simulink model "platoon_project"  (Simulink 8.9)
settings: Solver=FixedStepAuto  StartTime=0.0  StopTime=5  FixedStep=0.1  RelTol=1e-3  EnableMultiTasking=on
model workspace (MAT data in the model file):
  Kd_brake = 0
  Kd_throttle = 0
  Ki_brake = 1
  Ki_throttle = 1
  Kp_brake = 5000
  Kp_throttle = 15
  L : num (value not decoded)
values from neighbouring files (symbols this model uses):
  tnet_table = [57.5127074443 119.897368421 182.282029398 223.675296349 261.549751738 274.206057597 279.305263158 283.689473684 288.073684211 292.467532318 296.875779086 301.284025854 ... (400 elements, 20x20)]    [enginemap.mat]    (also in genmap.m = griddata(map_ford(:,1), map_ford(:,4), map_ford(:,2), we_tab)
  we_max = 471.2    [enginemap.mat]    (also in genmap.m = max(map_ford(:,1)))
  we_min = 57.6    [enginemap.mat]    (also in genmap.m = min(map_ford(:,1)))
undefined symbols (not defined in the file or in its folder): c_aero, delay_brake, F_roll, h, I_e, I_wheel, KB, mass, max_throttle, max_throttle_rate, min_throttle, mu_B, mu_C, mu_D, mu_E, P_po, Rdrive, tau_brake, tau_throttle, throttle_o, w_wheel_o, we_o, x_dot_o
libraries: simulink x10
(part 1 of 3)
settings Model: Creator=user  LastModifiedBy=edward
settings OptimizationCC: ExpressionDepthLimit=2147483647  InitFltsAndDblsToZero=on
settings DebuggingCC: SolverPrmCheckMsg=warning  FcnCallInpInsideContextMsg=error
settings GRTTargetCC: GeneratePreprocessorConditionals=Use local settings

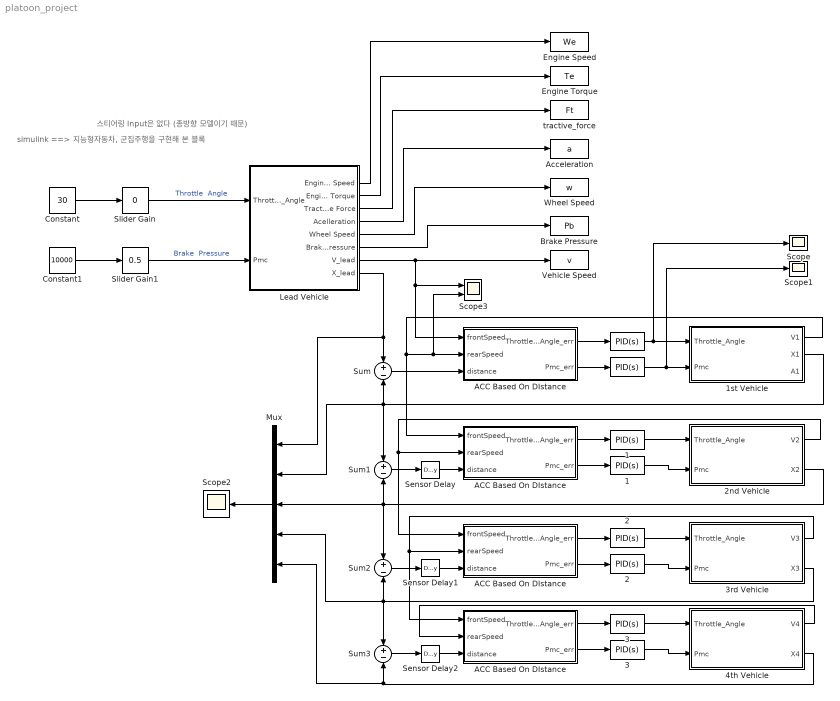
== system platoon_project ==
  note: simulink ==> 지능형자동차, 군집주행을 구현해 본 블록
  note: 스티어링 Input은 없다 (종방향 모델이기 때문)
   {,1..3} (4 alike) : simulink/Continuous/PID Controller  Controller=PID  TimeDomain=Continuous-time  SampleTime=-1  IntegratorMethod=Forward Euler  FilterMethod=Forward Euler  Form=Parallel  UseFilter=on  ControllerParametersSource=internal  P=Kp_throttle  I=Ki_throttle  D=Kd_throttle  N=100  InitialConditionSource=internal  InitialConditionForIntegrator=0  InitialConditionForFilter=0  ExternalReset=none  LimitOutput=off  UpperSaturationLimit=inf  LowerSaturationLimit=-inf  LinearizeAsGain=on  AntiWindupMode=none  Kb=1  TrackingMode=off  Kt=1  PParamMin=[]  PParamMax=[]  IParamMin=[]  IParamMax=[]  DParamMin=[]  DParamMax=[]  NParamMin=[]  NParamMax=[]  KbParamMin=[]  KbParamMax=[]  KtParamMin=[]  KtParamMax=[]  POutMin=[]  POutMax=[]  IOutMin=[]  IOutMax=[]  DOutMin=[]  DOutMax=[]  NOutMin=[]  NOutMax=[]  KbOutMin=[]  KbOutMax=[]  KtOutMin=[]  KtOutMax=[]  IntegratorOutMin=[]  IntegratorOutMax=[]  FilterOutMin=[]  FilterOutMax=[]  SumOutMin=[]  SumOutMax=[]  SumI1OutMin=[]  SumI1OutMax=[]  SumI2OutMin=[]  SumI2OutMax=[]  SumI3OutMin=[]  SumI3OutMax=[]  SumDOutMin=[]  SumDOutMax=[]  SaturationOutMin=[]  SaturationOutMax=[]  IntegratorContinuousStateAttributes=''  IntegratorStateMustResolveToSignalObject=off  IntegratorRTWStateStorageClass=Auto  FilterContinuousStateAttributes=''  FilterStateMustResolveToSignalObject=off  FilterRTWStateStorageClass=Auto  DifferentiatorICPrevScaledInput=0  DifferentiatorOutMin=[]  DifferentiatorOutMax=[]  InitialConditionSetting=State (most efficient)
    {,1..3} (4 alike) : simulink/Continuous/PID Controller  Controller=PID  TimeDomain=Continuous-time  SampleTime=-1  IntegratorMethod=Forward Euler  FilterMethod=Forward Euler  Form=Parallel  UseFilter=on  ControllerParametersSource=internal  P=Kp_brake  I=Ki_brake  D=Kd_brake  N=100  InitialConditionSource=internal  InitialConditionForIntegrator=0  InitialConditionForFilter=0  ExternalReset=none  LimitOutput=off  UpperSaturationLimit=inf  LowerSaturationLimit=-inf  LinearizeAsGain=on  AntiWindupMode=none  Kb=1  TrackingMode=off  Kt=1  PParamMin=[]  PParamMax=[]  IParamMin=[]  IParamMax=[]  DParamMin=[]  DParamMax=[]  NParamMin=[]  NParamMax=[]  KbParamMin=[]  KbParamMax=[]  KtParamMin=[]  KtParamMax=[]  POutMin=[]  POutMax=[]  IOutMin=[]  IOutMax=[]  DOutMin=[]  DOutMax=[]  NOutMin=[]  NOutMax=[]  KbOutMin=[]  KbOutMax=[]  KtOutMin=[]  KtOutMax=[]  IntegratorOutMin=[]  IntegratorOutMax=[]  FilterOutMin=[]  FilterOutMax=[]  SumOutMin=[]  SumOutMax=[]  SumI1OutMin=[]  SumI1OutMax=[]  SumI2OutMin=[]  SumI2OutMax=[]  SumI3OutMin=[]  SumI3OutMax=[]  SumDOutMin=[]  SumDOutMax=[]  SaturationOutMin=[]  SaturationOutMax=[]  IntegratorContinuousStateAttributes=''  IntegratorStateMustResolveToSignalObject=off  IntegratorRTWStateStorageClass=Auto  FilterContinuousStateAttributes=''  FilterStateMustResolveToSignalObject=off  FilterRTWStateStorageClass=Auto  DifferentiatorICPrevScaledInput=0  DifferentiatorOutMin=[]  DifferentiatorOutMax=[]  InitialConditionSetting=State (most efficient)
  "                ACC Based On DIstance           " : MATLAB Function  TreatAsAtomicUnit=on
  "               ACC Based On DIstance           " : MATLAB Function  TreatAsAtomicUnit=on
  "               ACC Based On DIstance            " : MATLAB Function  TreatAsAtomicUnit=on
  "               ACC Based On DIstance             " : MATLAB Function  TreatAsAtomicUnit=on
  1st Vehicle : Subsystem
  2nd Vehicle : Subsystem
  3rd Vehicle : Subsystem
  4th Vehicle : Subsystem
  Acceleration : ToWorkspace  VariableName=a  SampleTime=-1
  Brake Pressure : ToWorkspace  VariableName=Pb  SampleTime=-1
  Constant : Constant  Value=30
  Constant1 : Constant  Value=10000
  Engine Speed : ToWorkspace  VariableName=We  SampleTime=-1
  Engine Torque : ToWorkspace  VariableName=Te  SampleTime=-1
  Lead Vehicle : Subsystem
  Mux : Mux  Inputs=5
  Scope : Scope
  Scope1 : Scope
  Scope2 : Scope
  Scope3 : Scope  NumInputPorts=2
  Sensor Delay : TransportDelay  DelayTime=0.1
  Sensor Delay1 : TransportDelay  DelayTime=0.2
  Sensor Delay2 : TransportDelay  DelayTime=0.3
  Slider Gain : simulink/Math Operations/Slider Gain  gain=0  low=0  high=1
  Slider Gain1 : simulink/Math Operations/Slider Gain  gain=0.5  low=0  high=1
  Sum{,1..3} (4 alike) : Sum  Inputs=+|-
  Vehicle Speed : ToWorkspace  VariableName=v  SampleTime=-1
  Wheel Speed : ToWorkspace  VariableName=w  SampleTime=-1
  tractive_force : ToWorkspace  VariableName=Ft  SampleTime=-1
  wires:
  Constant/1 -> Slider Gain/1
  Slider Gain/1 -> Lead Vehicle/1(Throttle_Angle)  "Throttle  Angle"
  Constant1/1 -> Slider Gain1/1
  Slider Gain1/1 -> Lead Vehicle/2(Pmc)  "Brake  Pressure"
  Lead Vehicle/1(Engine Speed) -> Engine Speed/1
  Lead Vehicle/3(Tractive Force) -> tractive_force/1
  Lead Vehicle/4(Acelleration) -> Acceleration/1
  Lead Vehicle/5(Wheel Speed) -> Wheel Speed/1
  Lead Vehicle/6(Brake Pressure) -> Brake Pressure/1
  Lead Vehicle/2(Engine Torque) -> Engine Torque/1
  Lead Vehicle/8(X_lead) -> Mux/1, Sum/1
  1st Vehicle/2(X1) -> Mux/2, Sum1/1, Sum/2
  Sum/1 -> "               ACC Based On DIstance           "/3(distance)
  Lead Vehicle/7("V_lead ") -> "               ACC Based On DIstance           "/1(frontSpeed), Scope3/1, Vehicle Speed/1
  1st Vehicle/1(V1) -> "               ACC Based On DIstance            "/1(frontSpeed), Scope3/2, "               ACC Based On DIstance           "/2(rearSpeed)
  2nd Vehicle/2(X2) -> Mux/3, Sum2/1, Sum1/2
  2nd Vehicle/1(V2) -> "                ACC Based On DIstance           "/1(frontSpeed), "               ACC Based On DIstance            "/2(rearSpeed)
  Sum1/1 -> Sensor Delay/1
  "               ACC Based On DIstance           "/1(Throttle_Angle_err) -> " "/1
  "               ACC Based On DIstance           "/2(Pmc_err) -> "  "/1
  " "/1 -> Scope/1, 1st Vehicle/1(Throttle_Angle)
  " 1"/1 -> 2nd Vehicle/1(Throttle_Angle)
  "               ACC Based On DIstance            "/2(Pmc_err) -> "  1"/1
  "               ACC Based On DIstance            "/1(Throttle_Angle_err) -> " 1"/1
  "  1"/1 -> 2nd Vehicle/2(Pmc)
  "  2"/1 -> 3rd Vehicle/2(Pmc)
  " 2"/1 -> 3rd Vehicle/1(Throttle_Angle)
  "                ACC Based On DIstance           "/1(Throttle_Angle_err) -> " 2"/1
  "                ACC Based On DIstance           "/2(Pmc_err) -> "  2"/1
  " 3"/1 -> 4th Vehicle/1(Throttle_Angle)
  "  3"/1 -> 4th Vehicle/2(Pmc)
  "               ACC Based On DIstance             "/1(Throttle_Angle_err) -> " 3"/1
  "               ACC Based On DIstance             "/2(Pmc_err) -> "  3"/1
  3rd Vehicle/2(X3) -> Mux/4, Sum3/1, Sum2/2
  Sum2/1 -> Sensor Delay1/1
  3rd Vehicle/1(V3) -> "               ACC Based On DIstance             "/1(frontSpeed), "                ACC Based On DIstance           "/2(rearSpeed)
  4th Vehicle/2(X4) -> Mux/5, Sum3/2
  Sum3/1 -> Sensor Delay2/1
  4th Vehicle/1(V4) -> "               ACC Based On DIstance             "/2(rearSpeed)
  Sensor Delay/1 -> "               ACC Based On DIstance            "/3(distance)
  Sensor Delay1/1 -> "                ACC Based On DIstance           "/3(distance)
  Sensor Delay2/1 -> "               ACC Based On DIstance             "/3(distance)
  "  "/1 -> Scope1/1, 1st Vehicle/2(Pmc)
  Mux/1 -> Scope2/1

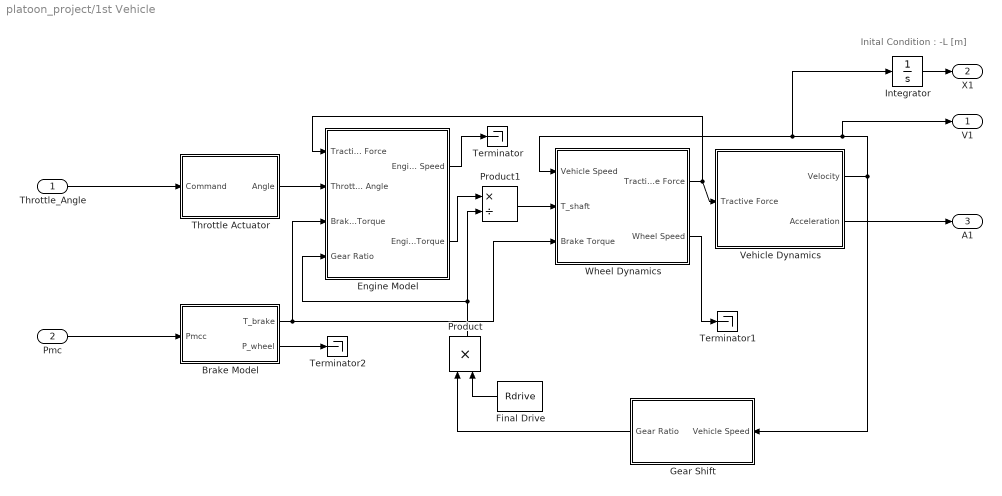
== system platoon_project/1st Vehicle ==
  note: Inital Condition : -L [m]
  Throttle_Angle : Inport
  Pmc : Inport  Port=2
  Brake Model : Subsystem
  Engine Model : Subsystem
  Final Drive : Constant  Value=Rdrive
  Gear Shift : Subsystem
  Integrator : Integrator  InitialCondition=-L
  Product : Product  Inputs=**  SaturateOnIntegerOverflow=on  RndMeth=Zero  InputSameDT=on  OutDataTypeStr=Inherit: Same as first input
  Product1 : Product  Inputs=*/  SaturateOnIntegerOverflow=on  RndMeth=Zero  InputSameDT=on  OutDataTypeStr=Inherit: Same as first input
  Terminator : Terminator
  Terminator1 : Terminator
  Terminator2 : Terminator
  Throttle Actuator : Subsystem
  Vehicle Dynamics : Subsystem
  Wheel Dynamics : Subsystem
  V1 : Outport
  X1 : Outport  Port=2
  A1 : Outport  Port=3
  wires:
  Vehicle Dynamics/1(Velocity) -> Gear Shift/1(Vehicle Speed), V1/1, Integrator/1, Wheel Dynamics/1(Vehicle Speed)
  Pmc/1 -> Brake Model/1(Pmcc)
  Throttle_Angle/1 -> Throttle Actuator/1(Command)
  Throttle Actuator/1(Angle) -> Engine Model/2(Throttle Angle)
  Wheel Dynamics/1(Tractive Force) -> Engine Model/1(Tractive Force), Vehicle Dynamics/1(Tractive Force)
  Gear Shift/1(Gear Ratio) -> Product/1
  Final Drive/1 -> Product/2
  Product/1 -> Engine Model/4(Gear Ratio), Product1/2
  Brake Model/1(T_brake) -> Wheel Dynamics/3(Brake Torque), Engine Model/3(Brake Torque)
  Engine Model/2(Engine Torque) -> Product1/1
  Product1/1 -> Wheel Dynamics/2(T_shaft)
  Engine Model/1(Engine Speed) -> Terminator/1
  Wheel Dynamics/2(Wheel Speed) -> Terminator1/1
  Brake Model/2(P_wheel) -> Terminator2/1
  Vehicle Dynamics/2(Acceleration) -> A1/1
  Integrator/1 -> X1/1

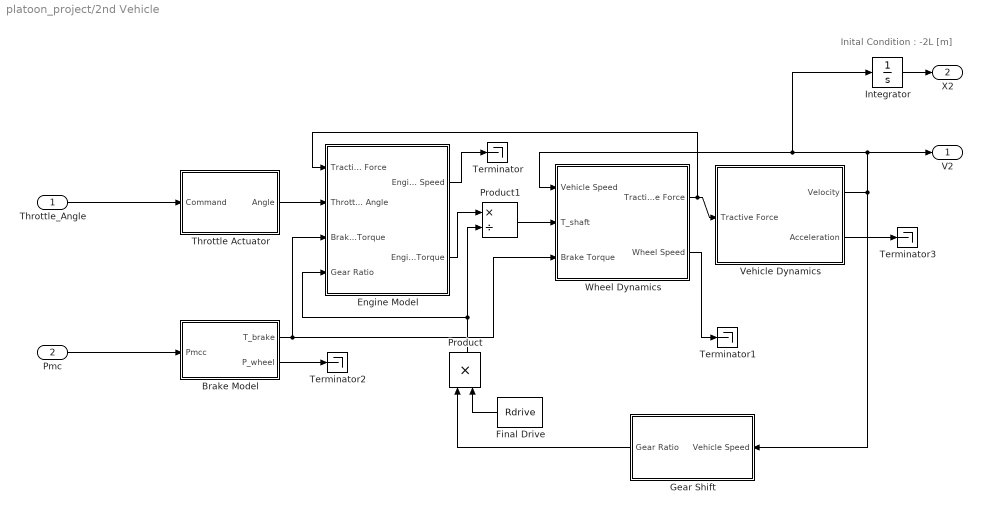
== system platoon_project/2nd Vehicle ==
  note: Inital Condition : -2L [m]
  Throttle_Angle : Inport
  Pmc : Inport  Port=2
  Brake Model : Subsystem
  Engine Model : Subsystem
  Final Drive : Constant  Value=Rdrive
  Gear Shift : Subsystem
  Integrator : Integrator  InitialCondition=-2*L
  Product : Product  Inputs=**  SaturateOnIntegerOverflow=on  RndMeth=Zero  InputSameDT=on  OutDataTypeStr=Inherit: Same as first input
  Product1 : Product  Inputs=*/  SaturateOnIntegerOverflow=on  RndMeth=Zero  InputSameDT=on  OutDataTypeStr=Inherit: Same as first input
  Terminator{,1..3} (4 alike) : Terminator
  Throttle Actuator : Subsystem
  Vehicle Dynamics : Subsystem
  Wheel Dynamics : Subsystem
  V2 : Outport
  X2 : Outport  Port=2
  wires:
  Integrator/1 -> X2/1
  Vehicle Dynamics/2(Acceleration) -> Terminator3/1
  Brake Model/2(P_wheel) -> Terminator2/1
  Wheel Dynamics/2(Wheel Speed) -> Terminator1/1
  Engine Model/1(Engine Speed) -> Terminator/1
  Product1/1 -> Wheel Dynamics/2(T_shaft)
  Engine Model/2(Engine Torque) -> Product1/1
  Brake Model/1(T_brake) -> Engine Model/3(Brake Torque), Wheel Dynamics/3(Brake Torque)
  Product/1 -> Product1/2, Engine Model/4(Gear Ratio)
  Final Drive/1 -> Product/2
  Gear Shift/1(Gear Ratio) -> Product/1
  Wheel Dynamics/1(Tractive Force) -> Vehicle Dynamics/1(Tractive Force), Engine Model/1(Tractive Force)
  Throttle Actuator/1(Angle) -> Engine Model/2(Throttle Angle)
  Throttle_Angle/1 -> Throttle Actuator/1(Command)
  Pmc/1 -> Brake Model/1(Pmcc)
  Vehicle Dynamics/1(Velocity) -> Wheel Dynamics/1(Vehicle Speed), Integrator/1, V2/1, Gear Shift/1(Vehicle Speed)

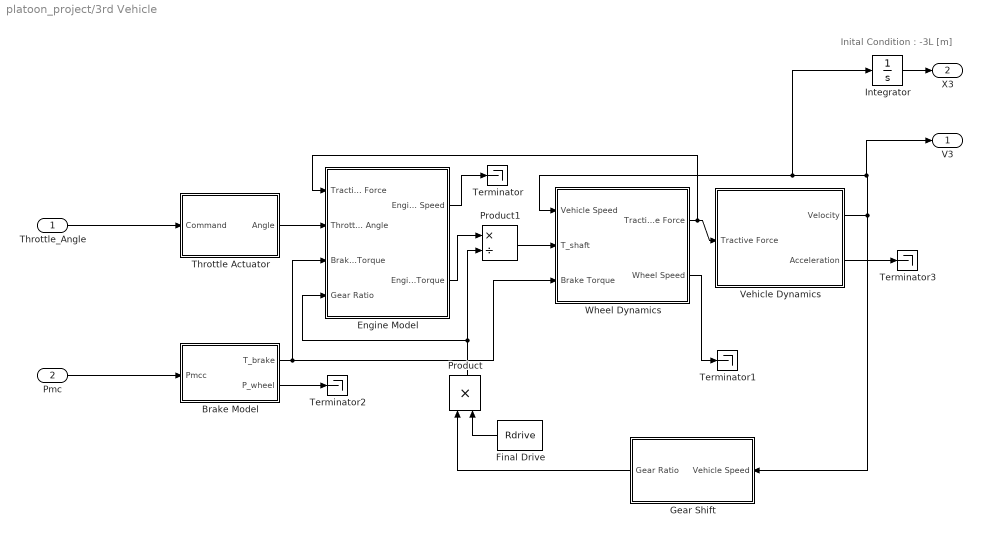
== system platoon_project/3rd Vehicle ==
  note: Inital Condition : -3L [m]
  Throttle_Angle : Inport
  Pmc : Inport  Port=2
  Brake Model : Subsystem
  Engine Model : Subsystem
  Final Drive : Constant  Value=Rdrive
  Gear Shift : Subsystem
  Integrator : Integrator  InitialCondition=-3*L
  Product : Product  Inputs=**  SaturateOnIntegerOverflow=on  RndMeth=Zero  InputSameDT=on  OutDataTypeStr=Inherit: Same as first input
  Product1 : Product  Inputs=*/  SaturateOnIntegerOverflow=on  RndMeth=Zero  InputSameDT=on  OutDataTypeStr=Inherit: Same as first input
  Terminator{,1..3} (4 alike) : Terminator
  Throttle Actuator : Subsystem
  Vehicle Dynamics : Subsystem
  Wheel Dynamics : Subsystem
  V3 : Outport
  X3 : Outport  Port=2
  wires:
  Pmc/1 -> Brake Model/1(Pmcc)
  Throttle_Angle/1 -> Throttle Actuator/1(Command)
  Throttle Actuator/1(Angle) -> Engine Model/2(Throttle Angle)
  Wheel Dynamics/1(Tractive Force) -> Engine Model/1(Tractive Force), Vehicle Dynamics/1(Tractive Force)
  Gear Shift/1(Gear Ratio) -> Product/1
  Final Drive/1 -> Product/2
  Product/1 -> Engine Model/4(Gear Ratio), Product1/2
  Brake Model/1(T_brake) -> Wheel Dynamics/3(Brake Torque), Engine Model/3(Brake Torque)
  Engine Model/2(Engine Torque) -> Product1/1
  Product1/1 -> Wheel Dynamics/2(T_shaft)
  Engine Model/1(Engine Speed) -> Terminator/1
  Wheel Dynamics/2(Wheel Speed) -> Terminator1/1
  Brake Model/2(P_wheel) -> Terminator2/1
  Vehicle Dynamics/2(Acceleration) -> Terminator3/1
  Integrator/1 -> X3/1
  Vehicle Dynamics/1(Velocity) -> Gear Shift/1(Vehicle Speed), V3/1, Integrator/1, Wheel Dynamics/1(Vehicle Speed)

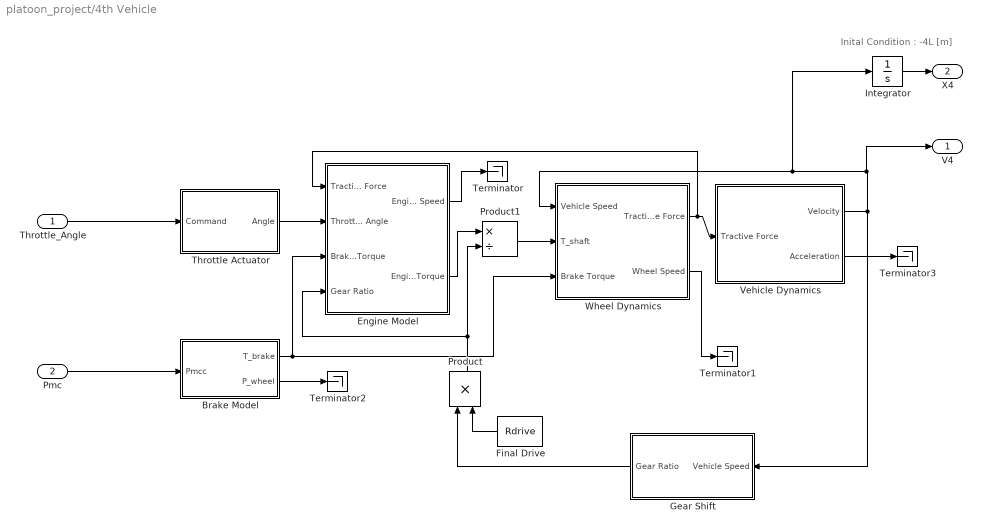
== system platoon_project/4th Vehicle ==
  note: Inital Condition : -4L [m]
  Throttle_Angle : Inport
  Pmc : Inport  Port=2
  Brake Model : Subsystem
  Engine Model : Subsystem
  Final Drive : Constant  Value=Rdrive
  Gear Shift : Subsystem
  Integrator : Integrator  InitialCondition=-4*L
  Product : Product  Inputs=**  SaturateOnIntegerOverflow=on  RndMeth=Zero  InputSameDT=on  OutDataTypeStr=Inherit: Same as first input
  Product1 : Product  Inputs=*/  SaturateOnIntegerOverflow=on  RndMeth=Zero  InputSameDT=on  OutDataTypeStr=Inherit: Same as first input
  Terminator{,1..3} (4 alike) : Terminator
  Throttle Actuator : Subsystem
  Vehicle Dynamics : Subsystem
  Wheel Dynamics : Subsystem
  V4 : Outport
  X4 : Outport  Port=2
  wires:
  Integrator/1 -> X4/1
  Vehicle Dynamics/2(Acceleration) -> Terminator3/1
  Brake Model/2(P_wheel) -> Terminator2/1
  Wheel Dynamics/2(Wheel Speed) -> Terminator1/1
  Engine Model/1(Engine Speed) -> Terminator/1
  Product1/1 -> Wheel Dynamics/2(T_shaft)
  Engine Model/2(Engine Torque) -> Product1/1
  Brake Model/1(T_brake) -> Engine Model/3(Brake Torque), Wheel Dynamics/3(Brake Torque)
  Product/1 -> Product1/2, Engine Model/4(Gear Ratio)
  Final Drive/1 -> Product/2
  Gear Shift/1(Gear Ratio) -> Product/1
  Wheel Dynamics/1(Tractive Force) -> Vehicle Dynamics/1(Tractive Force), Engine Model/1(Tractive Force)
  Throttle Actuator/1(Angle) -> Engine Model/2(Throttle Angle)
  Throttle_Angle/1 -> Throttle Actuator/1(Command)
  Pmc/1 -> Brake Model/1(Pmcc)
  Vehicle Dynamics/1(Velocity) -> V4/1, Wheel Dynamics/1(Vehicle Speed), Integrator/1, Gear Shift/1(Vehicle Speed)

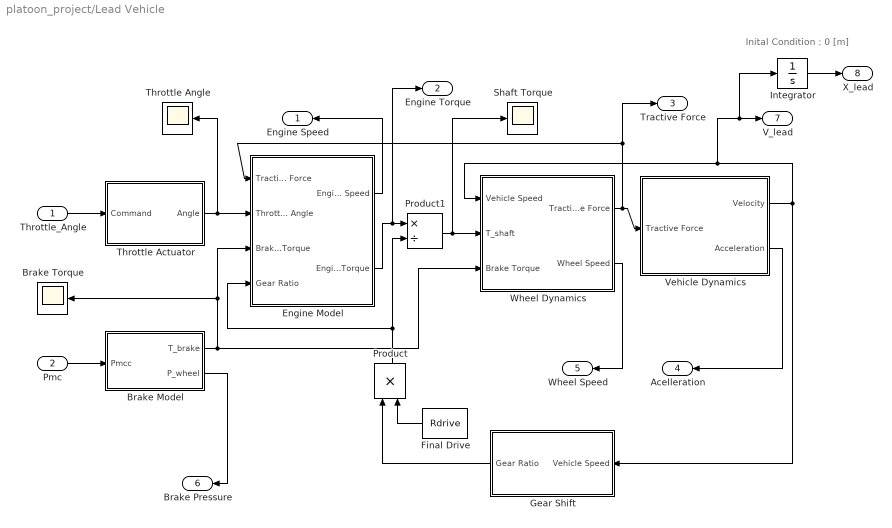
== system platoon_project/Lead Vehicle ==
  note: Inital Condition : 0 [m]
  Throttle_Angle : Inport
  Pmc : Inport  Port=2
  Brake Model : Subsystem
  Brake Torque : Scope
  Engine Model : Subsystem
  Final Drive : Constant  Value=Rdrive
  Gear Shift : Subsystem
  Integrator : Integrator
  Product : Product  Inputs=**  SaturateOnIntegerOverflow=on  RndMeth=Zero  InputSameDT=on  OutDataTypeStr=Inherit: Same as first input
  Product1 : Product  Inputs=*/  SaturateOnIntegerOverflow=on  RndMeth=Zero  InputSameDT=on  OutDataTypeStr=Inherit: Same as first input
  Shaft Torque : Scope
  Throttle Actuator : Subsystem
  Throttle Angle : Scope
  Vehicle Dynamics : Subsystem
  Wheel Dynamics : Subsystem
  Engine Speed : Outport
  Engine Torque : Outport  Port=2
  Tractive Force : Outport  Port=3
  Acelleration : Outport  Port=4
  Wheel Speed : Outport  Port=5
  Brake Pressure : Outport  Port=6
  "V_lead " : Outport  Port=7
  X_lead : Outport  Port=8
  wires:
  Product1/1 -> Shaft Torque/1, Wheel Dynamics/2(T_shaft)
  Engine Model/2(Engine Torque) -> Product1/1, Engine Torque/1
  Engine Model/1(Engine Speed) -> Engine Speed/1
  Brake Model/1(T_brake) -> Engine Model/3(Brake Torque), Brake Torque/1, Wheel Dynamics/3(Brake Torque)
  Product/1 -> Product1/2, Engine Model/4(Gear Ratio)
  Final Drive/1 -> Product/2
  Gear Shift/1(Gear Ratio) -> Product/1
  Wheel Dynamics/1(Tractive Force) -> Vehicle Dynamics/1(Tractive Force), Engine Model/1(Tractive Force), Tractive Force/1
  Throttle Actuator/1(Angle) -> Engine Model/2(Throttle Angle), Throttle Angle/1
  Throttle_Angle/1 -> Throttle Actuator/1(Command)
  Pmc/1 -> Brake Model/1(Pmcc)
  Brake Model/2(P_wheel) -> Brake Pressure/1
  Vehicle Dynamics/1(Velocity) -> Integrator/1, "V_lead "/1, Wheel Dynamics/1(Vehicle Speed), Gear Shift/1(Vehicle Speed)
  Vehicle Dynamics/2(Acceleration) -> Acelleration/1
  Wheel Dynamics/2(Wheel Speed) -> Wheel Speed/1
  Integrator/1 -> X_lead/1

== system platoon_project/1st Vehicle/Brake Model ==
  note: Valve를 여닫는 시간에 따라
      | 필연적으로 발생하는 Time Delay
  note: brake는 1차 전달함수의 response를 보인다
  note: Wheel pressure
  note: Wheel Pressure가 브레이크 패드에 있는
      | Spring(k)보다 크게 걸렸을 때에만 브레이크가 작동하므로
      | Dead Zone이 발생한다
  Pmcc : Inport
  Brake Coefficient : Gain  Gain=KB  SaturateOnIntegerOverflow=on  OutDataTypeStr=Inherit: Same as input  ParamDataTypeStr=Inherit: Same as input
  Brake Dynamics : TransferFcn  Denominator=[tau_brake 1]
  Dead Zone : DeadZone  LowerValue=-P_po  UpperValue=P_po  SaturateOnIntegerOverflow=on
  Pure Time Delay : TransportDelay  DelayTime=delay_brake
  T_brake : Outport
  P_wheel : Outport  Port=2
  wires:
  Pure Time Delay/1 -> Brake Dynamics/1
  Pmcc/1 -> Pure Time Delay/1
  Brake Dynamics/1 -> Dead Zone/1, P_wheel/1  "P_wheel"
  Dead Zone/1 -> Brake Coefficient/1
  Brake Coefficient/1 -> T_brake/1

== system platoon_project/1st Vehicle/Engine Model ==
  note: engine map이 저장되어있다
      | 2-D Lookup table
      |
      | input : Throttle angle, Engine speed
      | output : Engine torque
  Tractive Force : Inport
  Throttle Angle : Inport  Port=2
  Brake Torque : Inport  Port=3
  Gear Ratio : Inport  Port=4
  1/(I_e+4*I_w*R^2) : Fcn  Expr=u(1)/(I_e+4*I_wheel*u(2)^2)
  Integrator : Integrator  InitialCondition=we_o  LimitOutput=on  UpperSaturationLimit=[we_max]  LowerSaturationLimit=[we_min]
  Mux : Mux  Inputs=2
  Product : Product  SaturateOnIntegerOverflow=on  RndMeth=Zero  InputSameDT=on  OutDataTypeStr=Inherit: Same as first input
  Sum : Sum  Inputs=+|-  SaturateOnIntegerOverflow=on  InputSameDT=on  OutDataTypeStr=Inherit: Same as first input
  Sum1 : Sum  SaturateOnIntegerOverflow=on  InputSameDT=on  OutDataTypeStr=Inherit: Same as first input
  T_net : Lookup2D  RowIndex=alpha_table  ColumnIndex=we_table  Table=tnet_table  SaturateOnIntegerOverflow=on  InputSameDT=on
  wheel radius : Gain  Gain=h  Multiplication=Matrix(K*u)  SaturateOnIntegerOverflow=on  OutDataTypeStr=Inherit: Same as input  ParamDataTypeStr=Inherit: Same as input
  Engine Speed : Outport
  Engine Torque : Outport  Port=2
  wires:
  T_net/1 -> Sum/1, Engine Torque/1
  Mux/1 -> 1/(I_e+4*I_w*R^2)/1
  Sum/1 -> Mux/1
  Gear Ratio/1 -> Mux/2, Product/2
  Sum1/1 -> Product/1
  Product/1 -> Sum/2
  Brake Torque/1 -> Sum1/2
  wheel radius/1 -> Sum1/1
  Tractive Force/1 -> wheel radius/1
  1/(I_e+4*I_w*R^2)/1 -> Integrator/1  "w_dot"
  Integrator/1 -> T_net/2, Engine Speed/1  "w"
  Throttle Angle/1 -> T_net/1

== system platoon_project/1st Vehicle/Gear Shift ==
  note: 현재 차량 속도 vs 기어변속 속도를 비교한다
      | [0; 1; 1] 같은 [1,n]행렬이 반환된다
  note: [1 1 1]인 [n,1] 행렬과
      | 반환행렬을 곱해서
      | 스칼라값(기어값)을 만든다
  Vehicle Speed : Inport
  Convert m/s to mph : Gain  Gain=3.6/1.6  SaturateOnIntegerOverflow=on  OutDataTypeStr=Inherit: Same as input  ParamDataTypeStr=Inherit: Same as input
  Direct Look-Up of Gear ratio : LookupNDDirect  NumberOfTableDimensions=1  Table=[0.3423,0.6378,1.0,1.4184]
  Get gear-1 : Gain  Gain=ones(1,3)  Multiplication=Matrix(K*u)  SaturateOnIntegerOverflow=on  OutDataTypeStr=Inherit: Same as input  ParamDataTypeStr=Inherit: Same as input
  Relational Operator : RelationalOperator  Operator=>  RndMeth=Nearest  InputSameDT=on
  Shift Speeds : Constant  Value=[15 32 67]
  Gear Ratio : Outport
  wires:
  Direct Look-Up of Gear ratio/1 -> Gear Ratio/1
  Vehicle Speed/1 -> Convert m/s to mph/1
  Get gear-1/1 -> Direct Look-Up of Gear ratio/1
  Convert m/s to mph/1 -> Relational Operator/1
  Relational Operator/1 -> Get gear-1/1
  Shift Speeds/1 -> Relational Operator/2

== system platoon_project/1st Vehicle/Throttle Actuator ==
  Command : Inport
  Integrator : Integrator  InitialCondition=throttle_o  LimitOutput=on  UpperSaturationLimit=max_throttle  LowerSaturationLimit=min_throttle
  Saturation : Saturate  UpperLimit=max_throttle_rate  LowerLimit=-max_throttle_rate
  Sum : Sum  Inputs=-+|  SaturateOnIntegerOverflow=on  InputSameDT=on  OutDataTypeStr=Inherit: Same as first input
  Throttle Time Constant : Gain  Gain=1/tau_throttle  SaturateOnIntegerOverflow=on  OutDataTypeStr=Inherit: Same as input  ParamDataTypeStr=Inherit: Same as input
  Angle : Outport
  wires:
  Saturation/1 -> Integrator/1
  Throttle Time Constant/1 -> Saturation/1
  Sum/1 -> Throttle Time Constant/1
  Integrator/1 -> Sum/1, Angle/1
  Command/1 -> Sum/2

== system platoon_project/1st Vehicle/Vehicle Dynamics ==
  note: Initial Velocity = 21 [m/s]
  note: 구름저항 F_roll
  note: 공기저항 F_air
  note: v_dot
  note: v
  note: 타이어저항 F_road
  Tractive Force : Inport
  Aerodynamic Drag : Fcn  Expr=c_aero*u^2
  Divide by Mass : Gain  Gain=1/mass  Multiplication=Matrix(K*u)  SaturateOnIntegerOverflow=on  OutDataTypeStr=Inherit: Same as input  ParamDataTypeStr=Inherit: Same as input
  Integrator : Integrator  InitialCondition=x_dot_o  LimitOutput=on  LowerSaturationLimit=0
  Rolling Resistance : Constant  Value=F_roll
  Sum1 : Sum  Inputs=--+  SaturateOnIntegerOverflow=on  InputSameDT=on  OutDataTypeStr=Inherit: Same as first input
  Velocity : Outport
  Acceleration : Outport  Port=2
  wires:
  Aerodynamic Drag/1 -> Sum1/1
  Rolling Resistance/1 -> Sum1/2
  Sum1/1 -> Divide by Mass/1
  Integrator/1 -> Aerodynamic Drag/1, Velocity/1
  Divide by Mass/1 -> Integrator/1, Acceleration/1
  Tractive Force/1 -> Sum1/3

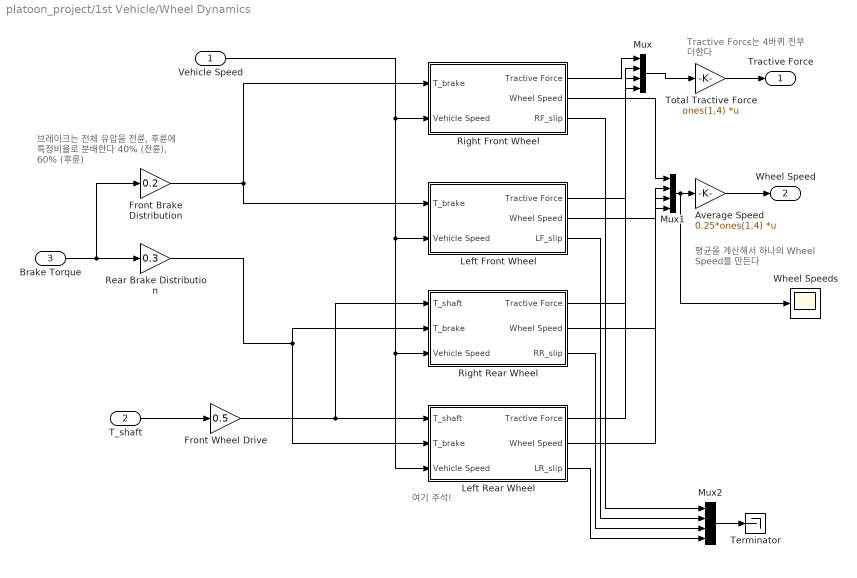
== system platoon_project/1st Vehicle/Wheel Dynamics ==
  note: 브레이크는 전체 유압을
      | 전륜, 후륜에 특정비율로 분배한다
      | 40% (전륜), 60% (후륜)
  note: 평균을 계산해서 하나의 Wheel Speed를 만든다
  note: Tractive Force는 4바퀴 전부 더한다
  note: 여기 주석!
  Vehicle Speed : Inport
  T_shaft : Inport  Port=2
  Brake Torque : Inport  Port=3
  Average Speed : Gain  Gain=0.25*ones(1,4)  Multiplication=Matrix(K*u)  SaturateOnIntegerOverflow=on  OutDataTypeStr=Inherit: Same as input  ParamDataTypeStr=Inherit: Same as input
  Front Brake Distribution : Gain  Gain=0.2  SaturateOnIntegerOverflow=on  OutDataTypeStr=Inherit: Same as input  ParamDataTypeStr=Inherit: Same as input
  Front Wheel Drive : Gain  Gain=0.5  SaturateOnIntegerOverflow=on  OutDataTypeStr=Inherit: Same as input  ParamDataTypeStr=Inherit: Same as input
  Left Front Wheel : Subsystem
  Left Rear Wheel : Subsystem
  Mux : Mux
  Mux1 : Mux
  Mux2 : Mux
  Rear Brake Distribution : Gain  Gain=0.3  SaturateOnIntegerOverflow=on  OutDataTypeStr=Inherit: Same as input  ParamDataTypeStr=Inherit: Same as input
  Right Front Wheel : Subsystem
  Right Rear Wheel : Subsystem
  Terminator : Terminator
  Total Tractive Force : Gain  Gain=ones(1,4)  Multiplication=Matrix(K*u)  SaturateOnIntegerOverflow=on  OutDataTypeStr=Inherit: Same as input  ParamDataTypeStr=Inherit: Same as input
  Wheel Speeds : Scope
  Tractive Force : Outport
  Wheel Speed : Outport  Port=2
  wires:
  Rear Brake Distribution/1 -> Right Rear Wheel/2(T_brake), Left Rear Wheel/2(T_brake)
  Front Brake Distribution/1 -> Left Front Wheel/1(T_brake), Right Front Wheel/1(T_brake)
  Right Rear Wheel/3(RR_slip) -> Mux2/3
  Left Front Wheel/3(LF_slip) -> Mux2/2
  Brake Torque/1 -> Front Brake Distribution/1, Rear Brake Distribution/1
  Front Wheel Drive/1 -> Left Rear Wheel/1(T_shaft), Right Rear Wheel/1(T_shaft)
  T_shaft/1 -> Front Wheel Drive/1
  Mux2/1 -> Terminator/1
  Left Rear Wheel/3(LR_slip) -> Mux2/4
  Right Front Wheel/3(RF_slip) -> Mux2/1
  Left Rear Wheel/2(Wheel Speed) -> Mux1/4
  Right Rear Wheel/2(Wheel Speed) -> Mux1/3
  Left Front Wheel/2(Wheel Speed) -> Mux1/2
  Right Front Wheel/2(Wheel Speed) -> Mux1/1
  Mux1/1 -> Wheel Speeds/1, Average Speed/1
  Left Rear Wheel/1(Tractive Force) -> Mux/4
  Right Rear Wheel/1(Tractive Force) -> Mux/3
  Left Front Wheel/1(Tractive Force) -> Mux/2
  Right Front Wheel/1(Tractive Force) -> Mux/1
  Vehicle Speed/1 -> Left Front Wheel/2(Vehicle Speed), Right Rear Wheel/3(Vehicle Speed), Left Rear Wheel/3(Vehicle Speed), Right Front Wheel/2(Vehicle Speed)
  Mux/1 -> Total Tractive Force/1
  Average Speed/1 -> Wheel Speed/1
  Total Tractive Force/1 -> Tractive Force/1

== system platoon_project/2nd Vehicle/Brake Model ==
  note: Wheel Pressure가 브레이크 패드에 있는
      | Spring(k)보다 크게 걸렸을 때에만 브레이크가 작동하므로
      | Dead Zone이 발생한다
  note: Wheel pressure
  note: brake는 1차 전달함수의 response를 보인다
  note: Valve를 여닫는 시간에 따라
      | 필연적으로 발생하는 Time Delay
  Pmcc : Inport
  Brake Coefficient : Gain  Gain=KB  SaturateOnIntegerOverflow=on  OutDataTypeStr=Inherit: Same as input  ParamDataTypeStr=Inherit: Same as input
  Brake Dynamics : TransferFcn  Denominator=[tau_brake 1]
  Dead Zone : DeadZone  LowerValue=-P_po  UpperValue=P_po  SaturateOnIntegerOverflow=on
  Pure Time Delay : TransportDelay  DelayTime=delay_brake
  T_brake : Outport
  P_wheel : Outport  Port=2
  wires:
  Brake Coefficient/1 -> T_brake/1
  Dead Zone/1 -> Brake Coefficient/1
  Brake Dynamics/1 -> P_wheel/1, Dead Zone/1  "P_wheel"
  Pmcc/1 -> Pure Time Delay/1
  Pure Time Delay/1 -> Brake Dynamics/1

== system platoon_project/2nd Vehicle/Engine Model ==
  note: engine map이 저장되어있다
      | 2-D Lookup table
      |
      | input : Throttle angle, Engine speed
      | output : Engine torque
  Tractive Force : Inport
  Throttle Angle : Inport  Port=2
  Brake Torque : Inport  Port=3
  Gear Ratio : Inport  Port=4
  1/(I_e+4*I_w*R^2) : Fcn  Expr=u(1)/(I_e+4*I_wheel*u(2)^2)
  Integrator : Integrator  InitialCondition=we_o  LimitOutput=on  UpperSaturationLimit=[we_max]  LowerSaturationLimit=[we_min]
  Mux : Mux  Inputs=2
  Product : Product  SaturateOnIntegerOverflow=on  RndMeth=Zero  InputSameDT=on  OutDataTypeStr=Inherit: Same as first input
  Sum : Sum  Inputs=+|-  SaturateOnIntegerOverflow=on  InputSameDT=on  OutDataTypeStr=Inherit: Same as first input
  Sum1 : Sum  SaturateOnIntegerOverflow=on  InputSameDT=on  OutDataTypeStr=Inherit: Same as first input
  T_net : Lookup2D  RowIndex=alpha_table  ColumnIndex=we_table  Table=tnet_table  SaturateOnIntegerOverflow=on  InputSameDT=on
  wheel radius : Gain  Gain=h  Multiplication=Matrix(K*u)  SaturateOnIntegerOverflow=on  OutDataTypeStr=Inherit: Same as input  ParamDataTypeStr=Inherit: Same as input
  Engine Speed : Outport
  Engine Torque : Outport  Port=2
  wires:
  Throttle Angle/1 -> T_net/1
  Integrator/1 -> Engine Speed/1, T_net/2  "w"
  1/(I_e+4*I_w*R^2)/1 -> Integrator/1  "w_dot"
  Tractive Force/1 -> wheel radius/1
  wheel radius/1 -> Sum1/1
  Brake Torque/1 -> Sum1/2
  Product/1 -> Sum/2
  Sum1/1 -> Product/1
  Gear Ratio/1 -> Product/2, Mux/2
  Sum/1 -> Mux/1
  Mux/1 -> 1/(I_e+4*I_w*R^2)/1
  T_net/1 -> Engine Torque/1, Sum/1

== system platoon_project/2nd Vehicle/Gear Shift ==
  note: [1 1 1]인 [n,1] 행렬과
      | 반환행렬을 곱해서
      | 스칼라값(기어값)을 만든다
  note: 현재 차량 속도 vs 기어변속 속도를 비교한다
      | [0; 1; 1] 같은 [1,n]행렬이 반환된다
  Vehicle Speed : Inport
  Convert m/s to mph : Gain  Gain=3.6/1.6  SaturateOnIntegerOverflow=on  OutDataTypeStr=Inherit: Same as input  ParamDataTypeStr=Inherit: Same as input
  Direct Look-Up of Gear ratio : LookupNDDirect  NumberOfTableDimensions=1  Table=[0.3423,0.6378,1.0,1.4184]
  Get gear-1 : Gain  Gain=ones(1,3)  Multiplication=Matrix(K*u)  SaturateOnIntegerOverflow=on  OutDataTypeStr=Inherit: Same as input  ParamDataTypeStr=Inherit: Same as input
  Relational Operator : RelationalOperator  Operator=>  RndMeth=Nearest  InputSameDT=on
  Shift Speeds : Constant  Value=[15 32 67]
  Gear Ratio : Outport
  wires:
  Shift Speeds/1 -> Relational Operator/2
  Relational Operator/1 -> Get gear-1/1
  Convert m/s to mph/1 -> Relational Operator/1
  Get gear-1/1 -> Direct Look-Up of Gear ratio/1
  Vehicle Speed/1 -> Convert m/s to mph/1
  Direct Look-Up of Gear ratio/1 -> Gear Ratio/1

== system platoon_project/2nd Vehicle/Throttle Actuator ==
  Command : Inport
  Integrator : Integrator  InitialCondition=throttle_o  LimitOutput=on  UpperSaturationLimit=max_throttle  LowerSaturationLimit=min_throttle
  Saturation : Saturate  UpperLimit=max_throttle_rate  LowerLimit=-max_throttle_rate
  Sum : Sum  Inputs=-+|  SaturateOnIntegerOverflow=on  InputSameDT=on  OutDataTypeStr=Inherit: Same as first input
  Throttle Time Constant : Gain  Gain=1/tau_throttle  SaturateOnIntegerOverflow=on  OutDataTypeStr=Inherit: Same as input  ParamDataTypeStr=Inherit: Same as input
  Angle : Outport
  wires:
  Command/1 -> Sum/2
  Integrator/1 -> Angle/1, Sum/1
  Sum/1 -> Throttle Time Constant/1
  Throttle Time Constant/1 -> Saturation/1
  Saturation/1 -> Integrator/1

== system platoon_project/2nd Vehicle/Vehicle Dynamics ==
  note: 타이어저항 F_road
  note: v
  note: v_dot
  note: 공기저항 F_air
  note: 구름저항 F_roll
  note: Initial Velocity = 21 [m/s]
  Tractive Force : Inport
  Aerodynamic Drag : Fcn  Expr=c_aero*u^2
  Divide by Mass : Gain  Gain=1/mass  Multiplication=Matrix(K*u)  SaturateOnIntegerOverflow=on  OutDataTypeStr=Inherit: Same as input  ParamDataTypeStr=Inherit: Same as input
  Integrator : Integrator  InitialCondition=x_dot_o  LimitOutput=on  LowerSaturationLimit=0
  Rolling Resistance : Constant  Value=F_roll
  Sum1 : Sum  Inputs=--+  SaturateOnIntegerOverflow=on  InputSameDT=on  OutDataTypeStr=Inherit: Same as first input
  Velocity : Outport
  Acceleration : Outport  Port=2
  wires:
  Tractive Force/1 -> Sum1/3
  Divide by Mass/1 -> Acceleration/1, Integrator/1
  Integrator/1 -> Velocity/1, Aerodynamic Drag/1
  Sum1/1 -> Divide by Mass/1
  Rolling Resistance/1 -> Sum1/2
  Aerodynamic Drag/1 -> Sum1/1

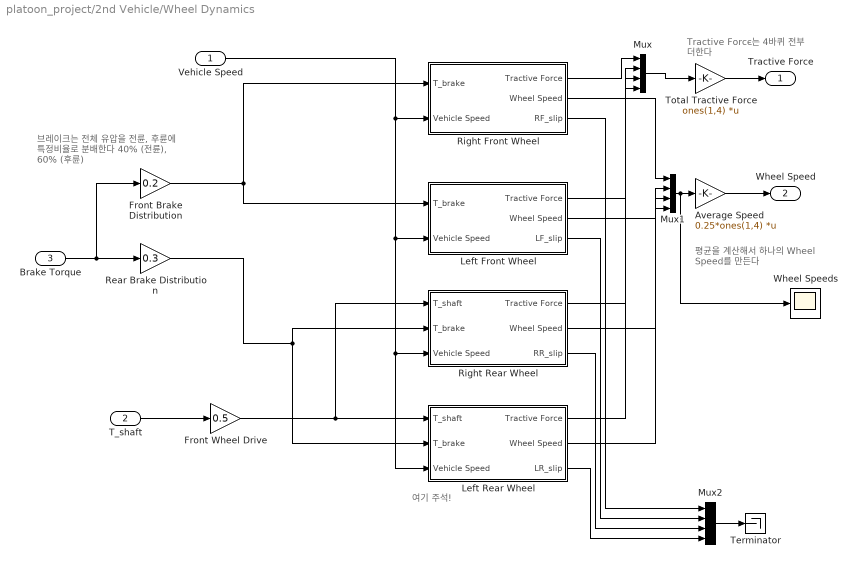
== system platoon_project/2nd Vehicle/Wheel Dynamics ==
  note: 여기 주석!
  note: Tractive Force는 4바퀴 전부 더한다
  note: 평균을 계산해서 하나의 Wheel Speed를 만든다
  note: 브레이크는 전체 유압을
      | 전륜, 후륜에 특정비율로 분배한다
      | 40% (전륜), 60% (후륜)
  Vehicle Speed : Inport
  T_shaft : Inport  Port=2
  Brake Torque : Inport  Port=3
  Average Speed : Gain  Gain=0.25*ones(1,4)  Multiplication=Matrix(K*u)  SaturateOnIntegerOverflow=on  OutDataTypeStr=Inherit: Same as input  ParamDataTypeStr=Inherit: Same as input
  Front Brake Distribution : Gain  Gain=0.2  SaturateOnIntegerOverflow=on  OutDataTypeStr=Inherit: Same as input  ParamDataTypeStr=Inherit: Same as input
  Front Wheel Drive : Gain  Gain=0.5  SaturateOnIntegerOverflow=on  OutDataTypeStr=Inherit: Same as input  ParamDataTypeStr=Inherit: Same as input
  Left Front Wheel : Subsystem
  Left Rear Wheel : Subsystem
  Mux : Mux
  Mux1 : Mux
  Mux2 : Mux
  Rear Brake Distribution : Gain  Gain=0.3  SaturateOnIntegerOverflow=on  OutDataTypeStr=Inherit: Same as input  ParamDataTypeStr=Inherit: Same as input
  Right Front Wheel : Subsystem
  Right Rear Wheel : Subsystem
  Terminator : Terminator
  Total Tractive Force : Gain  Gain=ones(1,4)  Multiplication=Matrix(K*u)  SaturateOnIntegerOverflow=on  OutDataTypeStr=Inherit: Same as input  ParamDataTypeStr=Inherit: Same as input
  Wheel Speeds : Scope
  Tractive Force : Outport
  Wheel Speed : Outport  Port=2
  wires:
  Total Tractive Force/1 -> Tractive Force/1
  Average Speed/1 -> Wheel Speed/1
  Mux/1 -> Total Tractive Force/1
  Vehicle Speed/1 -> Right Front Wheel/2(Vehicle Speed), Left Rear Wheel/3(Vehicle Speed), Right Rear Wheel/3(Vehicle Speed), Left Front Wheel/2(Vehicle Speed)
  Right Front Wheel/1(Tractive Force) -> Mux/1
  Left Front Wheel/1(Tractive Force) -> Mux/2
  Right Rear Wheel/1(Tractive Force) -> Mux/3
  Left Rear Wheel/1(Tractive Force) -> Mux/4
  Mux1/1 -> Average Speed/1, Wheel Speeds/1
  Right Front Wheel/2(Wheel Speed) -> Mux1/1
  Left Front Wheel/2(Wheel Speed) -> Mux1/2
  Right Rear Wheel/2(Wheel Speed) -> Mux1/3
  Left Rear Wheel/2(Wheel Speed) -> Mux1/4
  Right Front Wheel/3(RF_slip) -> Mux2/1
  Left Rear Wheel/3(LR_slip) -> Mux2/4
  Mux2/1 -> Terminator/1
  T_shaft/1 -> Front Wheel Drive/1
  Front Wheel Drive/1 -> Right Rear Wheel/1(T_shaft), Left Rear Wheel/1(T_shaft)
  Brake Torque/1 -> Rear Brake Distribution/1, Front Brake Distribution/1
  Left Front Wheel/3(LF_slip) -> Mux2/2
  Right Rear Wheel/3(RR_slip) -> Mux2/3
  Front Brake Distribution/1 -> Right Front Wheel/1(T_brake), Left Front Wheel/1(T_brake)
  Rear Brake Distribution/1 -> Left Rear Wheel/2(T_brake), Right Rear Wheel/2(T_brake)

== system platoon_project/3rd Vehicle/Brake Model ==
  note: Valve를 여닫는 시간에 따라
      | 필연적으로 발생하는 Time Delay
  note: brake는 1차 전달함수의 response를 보인다
  note: Wheel pressure
  note: Wheel Pressure가 브레이크 패드에 있는
      | Spring(k)보다 크게 걸렸을 때에만 브레이크가 작동하므로
      | Dead Zone이 발생한다
  Pmcc : Inport
  Brake Coefficient : Gain  Gain=KB  SaturateOnIntegerOverflow=on  OutDataTypeStr=Inherit: Same as input  ParamDataTypeStr=Inherit: Same as input
  Brake Dynamics : TransferFcn  Denominator=[tau_brake 1]
  Dead Zone : DeadZone  LowerValue=-P_po  UpperValue=P_po  SaturateOnIntegerOverflow=on
  Pure Time Delay : TransportDelay  DelayTime=delay_brake
  T_brake : Outport
  P_wheel : Outport  Port=2
  wires:
  Pure Time Delay/1 -> Brake Dynamics/1
  Pmcc/1 -> Pure Time Delay/1
  Brake Dynamics/1 -> Dead Zone/1, P_wheel/1  "P_wheel"
  Dead Zone/1 -> Brake Coefficient/1
  Brake Coefficient/1 -> T_brake/1

== system platoon_project/3rd Vehicle/Engine Model ==
  note: engine map이 저장되어있다
      | 2-D Lookup table
      |
      | input : Throttle angle, Engine speed
      | output : Engine torque
  Tractive Force : Inport
  Throttle Angle : Inport  Port=2
  Brake Torque : Inport  Port=3
  Gear Ratio : Inport  Port=4
  1/(I_e+4*I_w*R^2) : Fcn  Expr=u(1)/(I_e+4*I_wheel*u(2)^2)
  Integrator : Integrator  InitialCondition=we_o  LimitOutput=on  UpperSaturationLimit=[we_max]  LowerSaturationLimit=[we_min]
  Mux : Mux  Inputs=2
  Product : Product  SaturateOnIntegerOverflow=on  RndMeth=Zero  InputSameDT=on  OutDataTypeStr=Inherit: Same as first input
  Sum : Sum  Inputs=+|-  SaturateOnIntegerOverflow=on  InputSameDT=on  OutDataTypeStr=Inherit: Same as first input
  Sum1 : Sum  SaturateOnIntegerOverflow=on  InputSameDT=on  OutDataTypeStr=Inherit: Same as first input
  T_net : Lookup2D  RowIndex=alpha_table  ColumnIndex=we_table  Table=tnet_table  SaturateOnIntegerOverflow=on  InputSameDT=on
  wheel radius : Gain  Gain=h  Multiplication=Matrix(K*u)  SaturateOnIntegerOverflow=on  OutDataTypeStr=Inherit: Same as input  ParamDataTypeStr=Inherit: Same as input
  Engine Speed : Outport
  Engine Torque : Outport  Port=2
  wires:
  T_net/1 -> Sum/1, Engine Torque/1
  Mux/1 -> 1/(I_e+4*I_w*R^2)/1
  Sum/1 -> Mux/1
  Gear Ratio/1 -> Mux/2, Product/2
  Sum1/1 -> Product/1
  Product/1 -> Sum/2
  Brake Torque/1 -> Sum1/2
  wheel radius/1 -> Sum1/1
  Tractive Force/1 -> wheel radius/1
  1/(I_e+4*I_w*R^2)/1 -> Integrator/1  "w_dot"
  Integrator/1 -> T_net/2, Engine Speed/1  "w"
  Throttle Angle/1 -> T_net/1

== system platoon_project/3rd Vehicle/Gear Shift ==
  note: 현재 차량 속도 vs 기어변속 속도를 비교한다
      | [0; 1; 1] 같은 [1,n]행렬이 반환된다
  note: [1 1 1]인 [n,1] 행렬과
      | 반환행렬을 곱해서
      | 스칼라값(기어값)을 만든다
  Vehicle Speed : Inport
  Convert m/s to mph : Gain  Gain=3.6/1.6  SaturateOnIntegerOverflow=on  OutDataTypeStr=Inherit: Same as input  ParamDataTypeStr=Inherit: Same as input
  Direct Look-Up of Gear ratio : LookupNDDirect  NumberOfTableDimensions=1  Table=[0.3423,0.6378,1.0,1.4184]
  Get gear-1 : Gain  Gain=ones(1,3)  Multiplication=Matrix(K*u)  SaturateOnIntegerOverflow=on  OutDataTypeStr=Inherit: Same as input  ParamDataTypeStr=Inherit: Same as input
  Relational Operator : RelationalOperator  Operator=>  RndMeth=Nearest  InputSameDT=on
  Shift Speeds : Constant  Value=[15 32 67]
  Gear Ratio : Outport
  wires:
  Direct Look-Up of Gear ratio/1 -> Gear Ratio/1
  Vehicle Speed/1 -> Convert m/s to mph/1
  Get gear-1/1 -> Direct Look-Up of Gear ratio/1
  Convert m/s to mph/1 -> Relational Operator/1
  Relational Operator/1 -> Get gear-1/1
  Shift Speeds/1 -> Relational Operator/2

== system platoon_project/3rd Vehicle/Throttle Actuator ==
  Command : Inport
  Integrator : Integrator  InitialCondition=throttle_o  LimitOutput=on  UpperSaturationLimit=max_throttle  LowerSaturationLimit=min_throttle
  Saturation : Saturate  UpperLimit=max_throttle_rate  LowerLimit=-max_throttle_rate
  Sum : Sum  Inputs=-+|  SaturateOnIntegerOverflow=on  InputSameDT=on  OutDataTypeStr=Inherit: Same as first input
  Throttle Time Constant : Gain  Gain=1/tau_throttle  SaturateOnIntegerOverflow=on  OutDataTypeStr=Inherit: Same as input  ParamDataTypeStr=Inherit: Same as input
  Angle : Outport
  wires:
  Saturation/1 -> Integrator/1
  Throttle Time Constant/1 -> Saturation/1
  Sum/1 -> Throttle Time Constant/1
  Integrator/1 -> Sum/1, Angle/1
  Command/1 -> Sum/2

== system platoon_project/3rd Vehicle/Vehicle Dynamics ==
  note: 구름저항 F_roll
  note: 공기저항 F_air
  note: v_dot
  note: v
  note: 타이어저항 F_road
  note: Initial Velocity = 21 [m/s]
  Tractive Force : Inport
  Aerodynamic Drag : Fcn  Expr=c_aero*u^2
  Divide by Mass : Gain  Gain=1/mass  Multiplication=Matrix(K*u)  SaturateOnIntegerOverflow=on  OutDataTypeStr=Inherit: Same as input  ParamDataTypeStr=Inherit: Same as input
  Integrator : Integrator  InitialCondition=x_dot_o  LimitOutput=on  LowerSaturationLimit=0
  Rolling Resistance : Constant  Value=F_roll
  Sum1 : Sum  Inputs=--+  SaturateOnIntegerOverflow=on  InputSameDT=on  OutDataTypeStr=Inherit: Same as first input
  Velocity : Outport
  Acceleration : Outport  Port=2
  wires:
  Aerodynamic Drag/1 -> Sum1/1
  Rolling Resistance/1 -> Sum1/2
  Sum1/1 -> Divide by Mass/1
  Integrator/1 -> Aerodynamic Drag/1, Velocity/1
  Divide by Mass/1 -> Integrator/1, Acceleration/1
  Tractive Force/1 -> Sum1/3

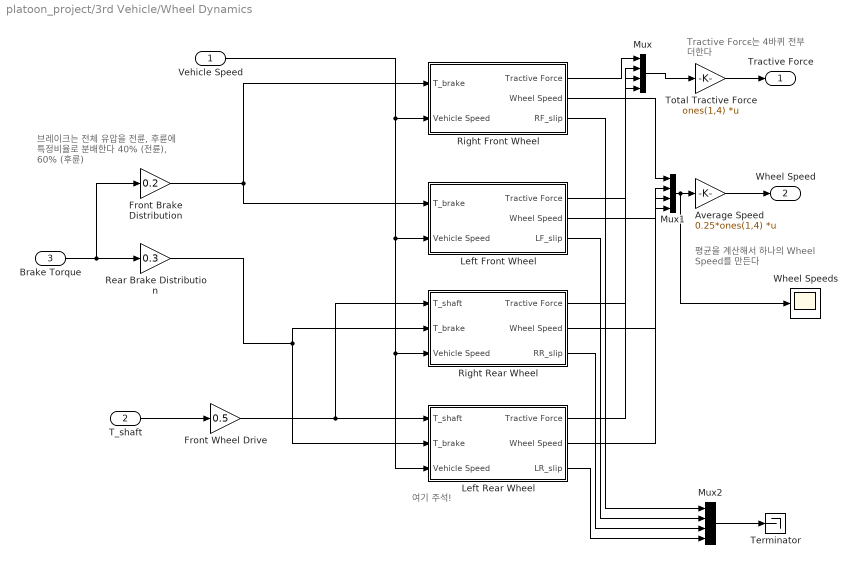
== system platoon_project/3rd Vehicle/Wheel Dynamics ==
  note: 브레이크는 전체 유압을
      | 전륜, 후륜에 특정비율로 분배한다
      | 40% (전륜), 60% (후륜)
  note: 평균을 계산해서 하나의 Wheel Speed를 만든다
  note: Tractive Force는 4바퀴 전부 더한다
  note: 여기 주석!
  Vehicle Speed : Inport
  T_shaft : Inport  Port=2
  Brake Torque : Inport  Port=3
  Average Speed : Gain  Gain=0.25*ones(1,4)  Multiplication=Matrix(K*u)  SaturateOnIntegerOverflow=on  OutDataTypeStr=Inherit: Same as input  ParamDataTypeStr=Inherit: Same as input
  Front Brake Distribution : Gain  Gain=0.2  SaturateOnIntegerOverflow=on  OutDataTypeStr=Inherit: Same as input  ParamDataTypeStr=Inherit: Same as input
  Front Wheel Drive : Gain  Gain=0.5  SaturateOnIntegerOverflow=on  OutDataTypeStr=Inherit: Same as input  ParamDataTypeStr=Inherit: Same as input
  Left Front Wheel : Subsystem
  Left Rear Wheel : Subsystem
  Mux : Mux
  Mux1 : Mux
  Mux2 : Mux
  Rear Brake Distribution : Gain  Gain=0.3  SaturateOnIntegerOverflow=on  OutDataTypeStr=Inherit: Same as input  ParamDataTypeStr=Inherit: Same as input
  Right Front Wheel : Subsystem
  Right Rear Wheel : Subsystem
  Terminator : Terminator
  Total Tractive Force : Gain  Gain=ones(1,4)  Multiplication=Matrix(K*u)  SaturateOnIntegerOverflow=on  OutDataTypeStr=Inherit: Same as input  ParamDataTypeStr=Inherit: Same as input
  Wheel Speeds : Scope
  Tractive Force : Outport
  Wheel Speed : Outport  Port=2
  wires:
  Rear Brake Distribution/1 -> Right Rear Wheel/2(T_brake), Left Rear Wheel/2(T_brake)
  Front Brake Distribution/1 -> Left Front Wheel/1(T_brake), Right Front Wheel/1(T_brake)
  Right Rear Wheel/3(RR_slip) -> Mux2/3
  Left Front Wheel/3(LF_slip) -> Mux2/2
  Brake Torque/1 -> Front Brake Distribution/1, Rear Brake Distribution/1
  Front Wheel Drive/1 -> Left Rear Wheel/1(T_shaft), Right Rear Wheel/1(T_shaft)
  T_shaft/1 -> Front Wheel Drive/1
  Mux2/1 -> Terminator/1
  Left Rear Wheel/3(LR_slip) -> Mux2/4
  Right Front Wheel/3(RF_slip) -> Mux2/1
  Left Rear Wheel/2(Wheel Speed) -> Mux1/4
  Right Rear Wheel/2(Wheel Speed) -> Mux1/3
  Left Front Wheel/2(Wheel Speed) -> Mux1/2
  Right Front Wheel/2(Wheel Speed) -> Mux1/1
  Mux1/1 -> Wheel Speeds/1, Average Speed/1
  Left Rear Wheel/1(Tractive Force) -> Mux/4
  Right Rear Wheel/1(Tractive Force) -> Mux/3
  Left Front Wheel/1(Tractive Force) -> Mux/2
  Right Front Wheel/1(Tractive Force) -> Mux/1
  Vehicle Speed/1 -> Left Front Wheel/2(Vehicle Speed), Right Rear Wheel/3(Vehicle Speed), Left Rear Wheel/3(Vehicle Speed), Right Front Wheel/2(Vehicle Speed)
  Mux/1 -> Total Tractive Force/1
  Average Speed/1 -> Wheel Speed/1
  Total Tractive Force/1 -> Tractive Force/1

== system platoon_project/4th Vehicle/Brake Model ==
  note: Wheel Pressure가 브레이크 패드에 있는
      | Spring(k)보다 크게 걸렸을 때에만 브레이크가 작동하므로
      | Dead Zone이 발생한다
  note: Wheel pressure
  note: brake는 1차 전달함수의 response를 보인다
  note: Valve를 여닫는 시간에 따라
      | 필연적으로 발생하는 Time Delay
  Pmcc : Inport
  Brake Coefficient : Gain  Gain=KB  SaturateOnIntegerOverflow=on  OutDataTypeStr=Inherit: Same as input  ParamDataTypeStr=Inherit: Same as input
  Brake Dynamics : TransferFcn  Denominator=[tau_brake 1]
  Dead Zone : DeadZone  LowerValue=-P_po  UpperValue=P_po  SaturateOnIntegerOverflow=on
  Pure Time Delay : TransportDelay  DelayTime=delay_brake
  T_brake : Outport
  P_wheel : Outport  Port=2
  wires:
  Brake Coefficient/1 -> T_brake/1
  Dead Zone/1 -> Brake Coefficient/1
  Brake Dynamics/1 -> P_wheel/1, Dead Zone/1  "P_wheel"
  Pmcc/1 -> Pure Time Delay/1
  Pure Time Delay/1 -> Brake Dynamics/1

== system platoon_project/4th Vehicle/Engine Model ==
  note: engine map이 저장되어있다
      | 2-D Lookup table
      |
      | input : Throttle angle, Engine speed
      | output : Engine torque
  Tractive Force : Inport
  Throttle Angle : Inport  Port=2
  Brake Torque : Inport  Port=3
  Gear Ratio : Inport  Port=4
  1/(I_e+4*I_w*R^2) : Fcn  Expr=u(1)/(I_e+4*I_wheel*u(2)^2)
  Integrator : Integrator  InitialCondition=we_o  LimitOutput=on  UpperSaturationLimit=[we_max]  LowerSaturationLimit=[we_min]
  Mux : Mux  Inputs=2
  Product : Product  SaturateOnIntegerOverflow=on  RndMeth=Zero  InputSameDT=on  OutDataTypeStr=Inherit: Same as first input
  Sum : Sum  Inputs=+|-  SaturateOnIntegerOverflow=on  InputSameDT=on  OutDataTypeStr=Inherit: Same as first input
  Sum1 : Sum  SaturateOnIntegerOverflow=on  InputSameDT=on  OutDataTypeStr=Inherit: Same as first input
  T_net : Lookup2D  RowIndex=alpha_table  ColumnIndex=we_table  Table=tnet_table  SaturateOnIntegerOverflow=on  InputSameDT=on
  wheel radius : Gain  Gain=h  Multiplication=Matrix(K*u)  SaturateOnIntegerOverflow=on  OutDataTypeStr=Inherit: Same as input  ParamDataTypeStr=Inherit: Same as input
  Engine Speed : Outport
  Engine Torque : Outport  Port=2
  wires:
  Throttle Angle/1 -> T_net/1
  Integrator/1 -> Engine Speed/1, T_net/2  "w"
  1/(I_e+4*I_w*R^2)/1 -> Integrator/1  "w_dot"
  Tractive Force/1 -> wheel radius/1
  wheel radius/1 -> Sum1/1
  Brake Torque/1 -> Sum1/2
  Product/1 -> Sum/2
  Sum1/1 -> Product/1
  Gear Ratio/1 -> Product/2, Mux/2
  Sum/1 -> Mux/1
  Mux/1 -> 1/(I_e+4*I_w*R^2)/1
  T_net/1 -> Engine Torque/1, Sum/1

== system platoon_project/4th Vehicle/Gear Shift ==
  note: [1 1 1]인 [n,1] 행렬과
      | 반환행렬을 곱해서
      | 스칼라값(기어값)을 만든다
  note: 현재 차량 속도 vs 기어변속 속도를 비교한다
      | [0; 1; 1] 같은 [1,n]행렬이 반환된다
  Vehicle Speed : Inport
  Convert m/s to mph : Gain  Gain=3.6/1.6  SaturateOnIntegerOverflow=on  OutDataTypeStr=Inherit: Same as input  ParamDataTypeStr=Inherit: Same as input
  Direct Look-Up of Gear ratio : LookupNDDirect  NumberOfTableDimensions=1  Table=[0.3423,0.6378,1.0,1.4184]
  Get gear-1 : Gain  Gain=ones(1,3)  Multiplication=Matrix(K*u)  SaturateOnIntegerOverflow=on  OutDataTypeStr=Inherit: Same as input  ParamDataTypeStr=Inherit: Same as input
  Relational Operator : RelationalOperator  Operator=>  RndMeth=Nearest  InputSameDT=on
  Shift Speeds : Constant  Value=[15 32 67]
  Gear Ratio : Outport
  wires:
  Shift Speeds/1 -> Relational Operator/2
  Relational Operator/1 -> Get gear-1/1
  Convert m/s to mph/1 -> Relational Operator/1
  Get gear-1/1 -> Direct Look-Up of Gear ratio/1
  Vehicle Speed/1 -> Convert m/s to mph/1
  Direct Look-Up of Gear ratio/1 -> Gear Ratio/1

== system platoon_project/4th Vehicle/Throttle Actuator ==
  Command : Inport
  Integrator : Integrator  InitialCondition=throttle_o  LimitOutput=on  UpperSaturationLimit=max_throttle  LowerSaturationLimit=min_throttle
  Saturation : Saturate  UpperLimit=max_throttle_rate  LowerLimit=-max_throttle_rate
  Sum : Sum  Inputs=-+|  SaturateOnIntegerOverflow=on  InputSameDT=on  OutDataTypeStr=Inherit: Same as first input
  Throttle Time Constant : Gain  Gain=1/tau_throttle  SaturateOnIntegerOverflow=on  OutDataTypeStr=Inherit: Same as input  ParamDataTypeStr=Inherit: Same as input
  Angle : Outport
  wires:
  Command/1 -> Sum/2
  Integrator/1 -> Angle/1, Sum/1
  Sum/1 -> Throttle Time Constant/1
  Throttle Time Constant/1 -> Saturation/1
  Saturation/1 -> Integrator/1

== system platoon_project/4th Vehicle/Vehicle Dynamics ==
  note: 타이어저항 F_road
  note: v
  note: v_dot
  note: 공기저항 F_air
  note: 구름저항 F_roll
  note: Initial Velocity = 21 [m/s]
  Tractive Force : Inport
  Aerodynamic Drag : Fcn  Expr=c_aero*u^2
  Divide by Mass : Gain  Gain=1/mass  Multiplication=Matrix(K*u)  SaturateOnIntegerOverflow=on  OutDataTypeStr=Inherit: Same as input  ParamDataTypeStr=Inherit: Same as input
  Integrator : Integrator  InitialCondition=x_dot_o  LimitOutput=on  LowerSaturationLimit=0
  Rolling Resistance : Constant  Value=F_roll
  Sum1 : Sum  Inputs=--+  SaturateOnIntegerOverflow=on  InputSameDT=on  OutDataTypeStr=Inherit: Same as first input
  Velocity : Outport
  Acceleration : Outport  Port=2
  wires:
  Tractive Force/1 -> Sum1/3
  Divide by Mass/1 -> Acceleration/1, Integrator/1
  Integrator/1 -> Velocity/1, Aerodynamic Drag/1
  Sum1/1 -> Divide by Mass/1
  Rolling Resistance/1 -> Sum1/2
  Aerodynamic Drag/1 -> Sum1/1

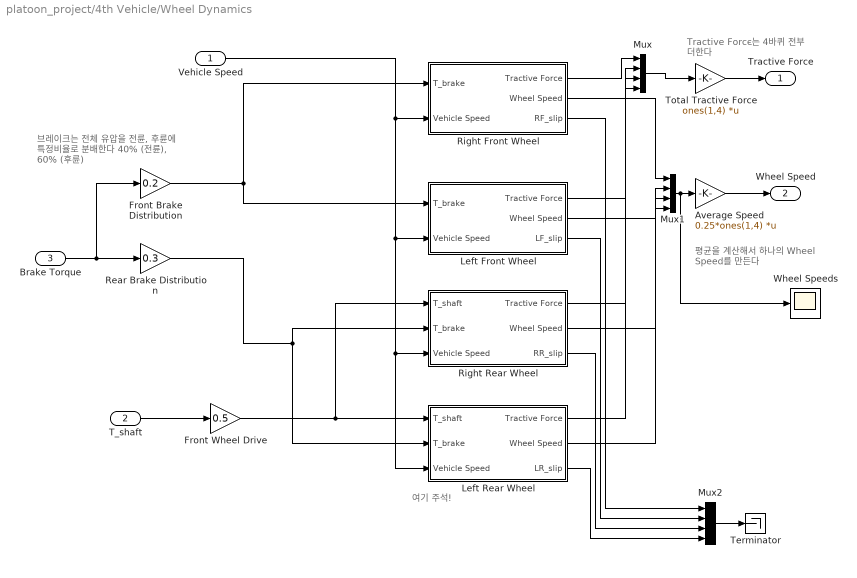
== system platoon_project/4th Vehicle/Wheel Dynamics ==
  note: 여기 주석!
  note: Tractive Force는 4바퀴 전부 더한다
  note: 평균을 계산해서 하나의 Wheel Speed를 만든다
  note: 브레이크는 전체 유압을
      | 전륜, 후륜에 특정비율로 분배한다
      | 40% (전륜), 60% (후륜)
  Vehicle Speed : Inport
  T_shaft : Inport  Port=2
  Brake Torque : Inport  Port=3
  Average Speed : Gain  Gain=0.25*ones(1,4)  Multiplication=Matrix(K*u)  SaturateOnIntegerOverflow=on  OutDataTypeStr=Inherit: Same as input  ParamDataTypeStr=Inherit: Same as input
  Front Brake Distribution : Gain  Gain=0.2  SaturateOnIntegerOverflow=on  OutDataTypeStr=Inherit: Same as input  ParamDataTypeStr=Inherit: Same as input
  Front Wheel Drive : Gain  Gain=0.5  SaturateOnIntegerOverflow=on  OutDataTypeStr=Inherit: Same as input  ParamDataTypeStr=Inherit: Same as input
  Left Front Wheel : Subsystem
  Left Rear Wheel : Subsystem
  Mux : Mux
  Mux1 : Mux
  Mux2 : Mux
  Rear Brake Distribution : Gain  Gain=0.3  SaturateOnIntegerOverflow=on  OutDataTypeStr=Inherit: Same as input  ParamDataTypeStr=Inherit: Same as input
  Right Front Wheel : Subsystem
  Right Rear Wheel : Subsystem
  Terminator : Terminator
  Total Tractive Force : Gain  Gain=ones(1,4)  Multiplication=Matrix(K*u)  SaturateOnIntegerOverflow=on  OutDataTypeStr=Inherit: Same as input  ParamDataTypeStr=Inherit: Same as input
  Wheel Speeds : Scope
  Tractive Force : Outport
  Wheel Speed : Outport  Port=2
  wires:
  Total Tractive Force/1 -> Tractive Force/1
  Average Speed/1 -> Wheel Speed/1
  Mux/1 -> Total Tractive Force/1
  Vehicle Speed/1 -> Right Front Wheel/2(Vehicle Speed), Left Rear Wheel/3(Vehicle Speed), Right Rear Wheel/3(Vehicle Speed), Left Front Wheel/2(Vehicle Speed)
  Right Front Wheel/1(Tractive Force) -> Mux/1
  Left Front Wheel/1(Tractive Force) -> Mux/2
  Right Rear Wheel/1(Tractive Force) -> Mux/3
  Left Rear Wheel/1(Tractive Force) -> Mux/4
  Mux1/1 -> Average Speed/1, Wheel Speeds/1
  Right Front Wheel/2(Wheel Speed) -> Mux1/1
  Left Front Wheel/2(Wheel Speed) -> Mux1/2
  Right Rear Wheel/2(Wheel Speed) -> Mux1/3
  Left Rear Wheel/2(Wheel Speed) -> Mux1/4
  Right Front Wheel/3(RF_slip) -> Mux2/1
  Left Rear Wheel/3(LR_slip) -> Mux2/4
  Mux2/1 -> Terminator/1
  T_shaft/1 -> Front Wheel Drive/1
  Front Wheel Drive/1 -> Right Rear Wheel/1(T_shaft), Left Rear Wheel/1(T_shaft)
  Brake Torque/1 -> Rear Brake Distribution/1, Front Brake Distribution/1
  Left Front Wheel/3(LF_slip) -> Mux2/2
  Right Rear Wheel/3(RR_slip) -> Mux2/3
  Front Brake Distribution/1 -> Right Front Wheel/1(T_brake), Left Front Wheel/1(T_brake)
  Rear Brake Distribution/1 -> Left Rear Wheel/2(T_brake), Right Rear Wheel/2(T_brake)

== system platoon_project/Lead Vehicle/Brake Model ==
  note: Wheel Pressure가 브레이크 패드에 있는
      | Spring(k)보다 크게 걸렸을 때에만 브레이크가 작동하므로
      | Dead Zone이 발생한다
  note: Wheel pressure
  note: brake는 1차 전달함수의 response를 보인다
  note: Valve를 여닫는 시간에 따라
      | 필연적으로 발생하는 Time Delay
  Pmcc : Inport
  Brake Coefficient : Gain  Gain=KB  SaturateOnIntegerOverflow=on  OutDataTypeStr=Inherit: Same as input  ParamDataTypeStr=Inherit: Same as input
  Brake Dynamics : TransferFcn  Denominator=[tau_brake 1]
  Dead Zone : DeadZone  LowerValue=-P_po  UpperValue=P_po  SaturateOnIntegerOverflow=on
  Pure Time Delay : TransportDelay  DelayTime=delay_brake
  T_brake : Outport
  P_wheel : Outport  Port=2
  wires:
  Brake Coefficient/1 -> T_brake/1
  Dead Zone/1 -> Brake Coefficient/1
  Brake Dynamics/1 -> P_wheel/1, Dead Zone/1  "P_wheel"
  Pmcc/1 -> Pure Time Delay/1
  Pure Time Delay/1 -> Brake Dynamics/1
